simulink model "SOC_Estimation_EKF"  (R2025b)
settings: Solver=FixedStepDiscrete  StartTime=0.0  StopTime=10000  FixedStep=0.1  RelTol=1e-3
model workspace (MAT data in the model file):
  R = 20
  Rmn = 0.0008432
  Ts = 0.2
libraries: BatteryEstimators x1
settings Model: Creator=HP  LastModifiedBy=HP

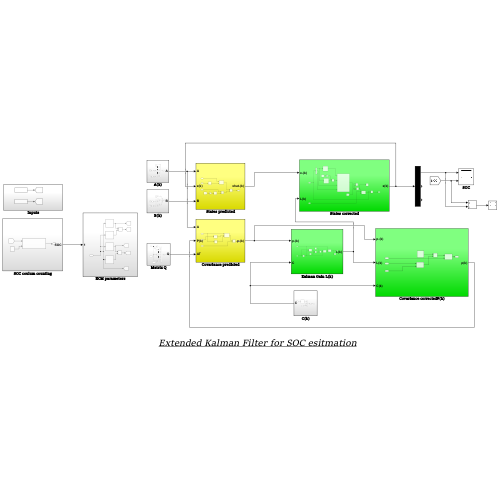
[thumbnail: Simulink's stored preview of the top-level diagram]
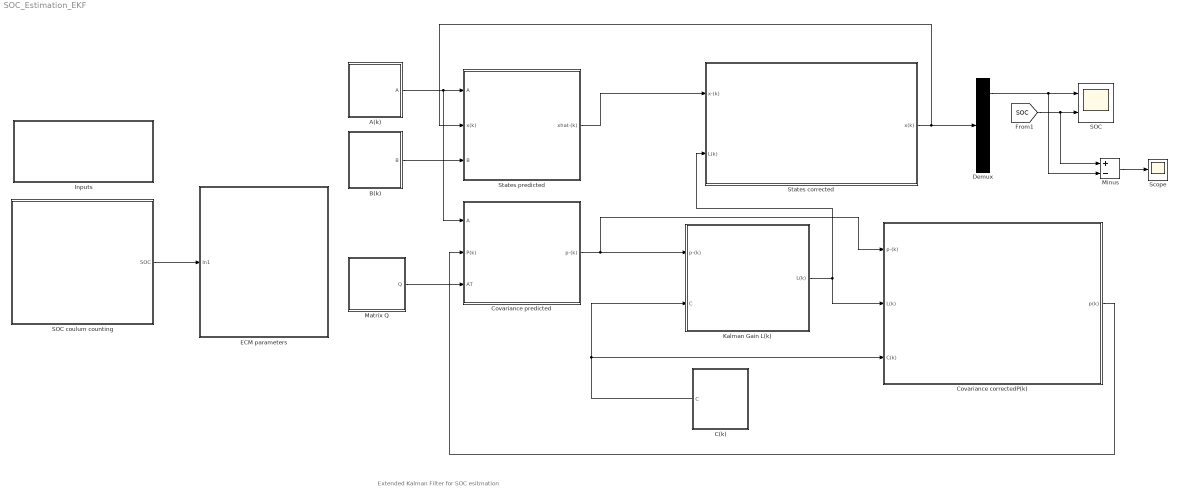
== system SOC_Estimation_EKF ==
  note: Extended Kalman Filter for SOC esitmation
  A(k) : Subsystem
  B(k) : Subsystem
  C(k) : Subsystem
  Covariance correctedP(k) : Subsystem
  Covariance predicted : Subsystem
  Demux : Demux  Outputs=3
  ECM parameters : Subsystem
  Inputs : Subsystem
  Kalman Gain L(k) : Subsystem
  Matrix Q : Subsystem
  Minus : Sum  Inputs=+-
  SOC : Scope  NumInputPorts=2
      settings: ActiveDisplayYMinimum=-0.11556307804743458  ActiveDisplayYMaximum=1.1239514531163817
  SOC coulum counting : Subsystem
  Scope : Scope
      settings: ActiveDisplayYMinimum=-0.040133146008147769  ActiveDisplayYMaximum=0.033848860038154627  DataLoggingVariableName=ScopeData4
  States corrected : Subsystem
  States predicted : Subsystem
  wires:
  A(k)/1(A) -> States predicted/1(A), Covariance predicted/1(A)
  B(k)/1(B) -> States predicted/3(B)
  Matrix Q/1(Q) -> Covariance predicted/3(AT)
  Covariance predicted/1(p-(k)) -> Kalman Gain L(k)/1(p-(k)), Covariance correctedP(k)/1(p-(k))
  C(k)/1(C) -> Kalman Gain L(k)/2(C), Covariance correctedP(k)/3(C(k))
  Kalman Gain L(k)/1(L(k)) -> States corrected/2(L(k)), Covariance correctedP(k)/2(L(k))
  Covariance correctedP(k)/1(p(k)) -> Covariance predicted/2(P(k))
  States predicted/1(xhat-(k)) -> States corrected/1(x-(k))
  States corrected/1(x(k)) -> States predicted/2(x(k)), Demux/1
  Demux/1 -> Minus/2, SOC/1
  [SOC] -> Minus/1, SOC/2
  SOC coulum counting/1(SOC) -> ECM parameters/1(In1)
  Minus/1 -> Scope/1

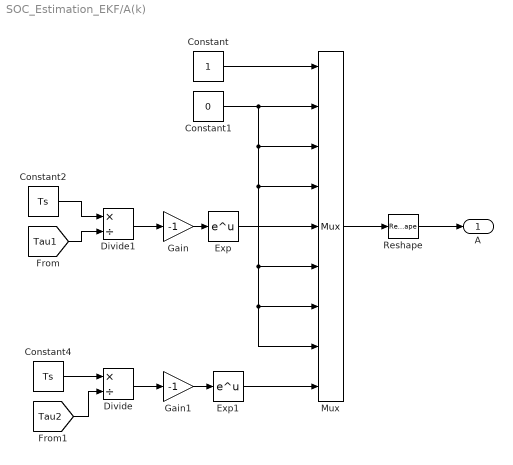
== system SOC_Estimation_EKF/A(k) ==
  Constant : Constant
  Constant1 : Constant  Value=0
  Constant2 : Constant  Value=Ts
  Constant4 : Constant  Value=Ts
  Divide : Product  Inputs=*/
  Divide1 : Product  Inputs=*/
  Exp : Math
  Exp1 : Math
  Gain : Gain  Gain=-1
  Gain1 : Gain  Gain=-1
  Mux : Mux  Inputs=9
  Reshape : Reshape  OutputDimensionality=Customize  OutputDimensions=[3,3]
  A : Outport
  wires:
  Constant1/1 -> Mux/6, Mux/7, Mux/8, Mux/4, Mux/3, Mux/2
  Constant4/1 -> Divide/1
  Constant/1 -> Mux/1
  [Tau2] -> Divide/2
  Divide1/1 -> Gain/1
  Gain1/1 -> Exp1/1
  Gain/1 -> Exp/1
  Divide/1 -> Gain1/1
  Constant2/1 -> Divide1/1
  [Tau1] -> Divide1/2
  Mux/1 -> Reshape/1
  Reshape/1 -> A/1
  Exp/1 -> Mux/5
  Exp1/1 -> Mux/9

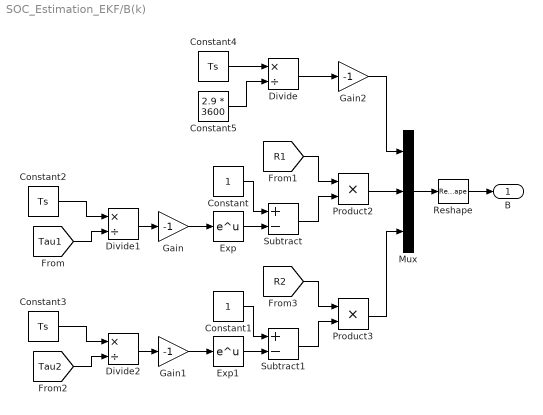
== system SOC_Estimation_EKF/B(k) ==
  Constant : Constant
  Constant1 : Constant
  Constant2 : Constant  Value=Ts
  Constant3 : Constant  Value=Ts
  Constant4 : Constant  Value=Ts
  Constant5 : Constant  Value=2.9 * 3600
  Divide : Product  Inputs=*/
  Divide1 : Product  Inputs=*/
  Divide2 : Product  Inputs=*/
  Exp : Math
  Exp1 : Math
  Gain : Gain  Gain=-1
  Gain1 : Gain  Gain=-1
  Gain2 : Gain  Gain=-1
  Mux : Mux  Inputs=3
  Product2 : Product
  Product3 : Product
  Reshape : Reshape  OutputDimensionality=Customize  OutputDimensions=[3,1]
  Subtract : Sum  Inputs=+-
  Subtract1 : Sum  Inputs=+-
  B : Outport
  wires:
  Product3/1 -> Mux/3
  Gain/1 -> Exp/1
  Constant3/1 -> Divide2/1
  [R2] -> Product3/1
  Constant/1 -> Subtract/1
  Divide/1 -> Gain2/1
  Gain2/1 -> Mux/1
  Subtract1/1 -> Product3/2
  Divide2/1 -> Gain1/1
  [Tau2] -> Divide2/2
  Gain1/1 -> Exp1/1
  Constant1/1 -> Subtract1/1
  Constant5/1 -> Divide/2
  Exp1/1 -> Subtract1/2
  Constant2/1 -> Divide1/1
  [Tau1] -> Divide1/2
  Divide1/1 -> Gain/1
  [R1] -> Product2/1
  Constant4/1 -> Divide/1
  Product2/1 -> Mux/2
  Subtract/1 -> Product2/2
  Mux/1 -> Reshape/1
  Exp/1 -> Subtract/2
  Reshape/1 -> B/1

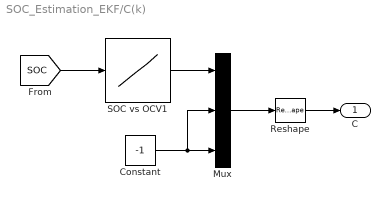
== system SOC_Estimation_EKF/C(k) ==
  Constant : Constant  Value=-1
  Mux : Mux  Inputs=3
  Reshape : Reshape  OutputDimensionality=Customize  OutputDimensions=[1,3]
  SOC vs OCV1 : Lookup_n-D  NumberOfTableDimensions=1  BreakpointsForDimension1=[0;0.017000000000000001;0.034000000000000002;0.050999999999999997;0.068000000000000005;0.085000000000000006;0.10199999999999999;0.11899999999999999;0.13600000000000001;0.152;0.16900000000000001;0.186;0.20300000000000001;0.22;0.23699999999999999;0.254;0.27100000000000002;0.28799999999999998;0.30499999999999999;0.32200000000000001;0.33900000000000002;0.35599999999999998;0.373;0.39000000000000001;0.40699999999999997;0.42399999999999999;0.441;0.45800000000000002;0.47499999999999998;0.49199999999999999;0.50800000000000001;0.52500000000000002;0.54200000000000004;0.55900000000000005;0.57599999999999996;0.59299999999999997;0.60999999999999999;0.627;0.64400000000000002;0.66100000000000003;0.67800000000000005;0.69499999999999995;0.71199999999999997;0.72899999999999998;0.746;0.76300000000000001;0.78000000000000003;0.79700000000000004;0.81399999999999995;0.82999999999999996;0.84699999999999998;0.86399999999999999;0.88100000000000001;0.89800000000000002;0.91500000000000004;0.93200000000000005;0.94899999999999995;0.96599999999999997;0.98299999999999998;1]  BreakpointsForDimension3=[5, 7]  Table=[32.28235294;20.56764706;6.15294118;2.68235294;1.62647059;1.24705882;1.28529412;1.43823529;1.42352941;1.32647059;1.17352941;1.05882353;1.05882353;1.00588235;0.89117647;0.79411765;0.71764706;0.66176471;0.60588235;0.56764706;0.56764706;0.56764706;0.5470588199999999;0.56764706;0.56764706;0.56764706;0.58823529;0.66176471;0.6882352900000001;0.67352941;0.7647058799999999;0.89117647;1.02352941;1.13823529;1.17352941;1.10882353;0.99117647;0.94705882;0.90882353;0.86470588;0.8441176500000001;0.83235294;0.81470588;0.79411765;0.79411765;0.82352941;0.90882353;0.97352941;1.00588235;1.02058824;1.11764706;1.22647059;1.10294118;0.97941176;0.87352941;0.79411765;0.79411765;1.00588235;1.30294118;1.4]  InternalRulePriority=Speed  RndMeth=Simplest
  C : Outport
  wires:
  SOC vs OCV1/1 -> Mux/1
  Constant/1 -> Mux/2, Mux/3
  [SOC] -> SOC vs OCV1/1
  Mux/1 -> Reshape/1
  Reshape/1 -> C/1

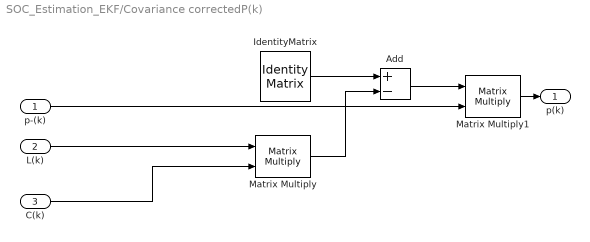
== system SOC_Estimation_EKF/Covariance correctedP(k) ==
  p-(k) : Inport
  L(k) : Inport  Port=2
  C(k) : Inport  Port=3
  Add : Sum  Inputs=+-
  IdentityMatrix : IdentityMatrix  OutputDimensions=3
  Matrix Multiply : Product  Multiplication=Matrix(*)
  Matrix Multiply1 : Product  Multiplication=Matrix(*)
  p(k) : Outport
  wires:
  Matrix Multiply/1 -> Add/2
  L(k)/1 -> Matrix Multiply/1
  p-(k)/1 -> Matrix Multiply1/2
  C(k)/1 -> Matrix Multiply/2
  IdentityMatrix/1 -> Add/1
  Add/1 -> Matrix Multiply1/1
  Matrix Multiply1/1 -> p(k)/1

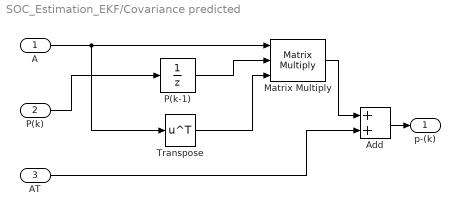
== system SOC_Estimation_EKF/Covariance predicted ==
  A : Inport
  P(k) : Inport  Port=2
  AT : Inport  Port=3
  Add : Sum
  Matrix Multiply : Product  Inputs=3  Multiplication=Matrix(*)
  P(k-1) : UnitDelay  SampleTime=-1  HasFrameUpgradeWarning=on
  Transpose : Math  Operator=transpose
  p-(k) : Outport
  wires:
  P(k)/1 -> P(k-1)/1
  A/1 -> Matrix Multiply/1, Transpose/1
  P(k-1)/1 -> Matrix Multiply/2
  AT/1 -> Add/2
  Transpose/1 -> Matrix Multiply/3
  Add/1 -> p-(k)/1
  Matrix Multiply/1 -> Add/1

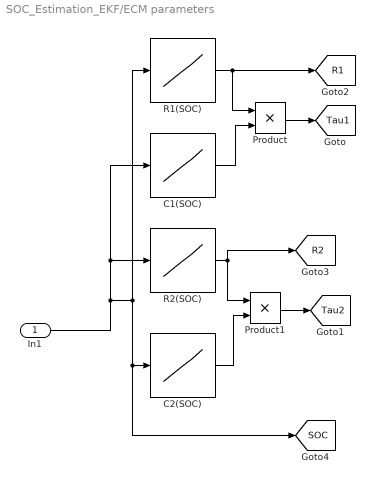
== system SOC_Estimation_EKF/ECM parameters ==
  In1 : Inport
  C1(SOC) : Lookup_n-D  NumberOfTableDimensions=1  BreakpointsForDimension1=[0.045807;0.04861;0.049997;0.09027200000000001;0.095828;0.098607;0.099993;0.14024;0.1458;0.14861;0.15;0.17914;0.19025;0.1958;0.19861;0.19999;0.22914;0.24025;0.24581;0.24861;0.25;0.27914;0.29025;0.29581;0.29861;0.3;0.37915;0.39027;0.39583;0.3986;0.39999;0.47914;0.49025;0.4958;0.49861;0.49999;0.57917;0.59027;0.59583;0.59861;0.67913;0.69025;0.69581;0.69861;0.7;0.7791400000000001;0.79025;0.79581;0.79861;0.8;0.87904;0.8902600000000001;0.8958199999999999;0.8986;0.9;0.92903;0.94025;0.94581;0.94861;0.95;0.97914;0.99026;0.99581;0.99861;1]  BreakpointsForDimension3=[5, 7]  Table=[9.757899999999999;10.71;19.27;9.6311;10.157;9.1839;7.5693;15.897;6.3554;7.6236;6.7393;7.7947;34.343;7.0897;6.9869;8.0646;10.291;128.49;9.2583;8.628;10.569;3.0789;34.161;8.1753;8.1843;13.019;10.1;46.123;9.795400000000001;11.091;15.634;8.213800000000001;31.921;9.789999999999999;10.357;12.364;15.812;507.21;15.291;17.025;4.9769;86.715;10.771;11.678;16.952;4.0064;71.312;13.377;14.851;17.855;16.185;258.83;9.310700000000001;12.325;12.739;12.404;193.01;11.32;10.578;11.323;10.955;21.418;8.9283;8.207800000000001;7.1378]  InternalRulePriority=Speed  RndMeth=Simplest
  C2(SOC) : Lookup_n-D  NumberOfTableDimensions=1  BreakpointsForDimension1=[0.045807;0.04861;0.049997;0.09027200000000001;0.095828;0.098607;0.099993;0.14024;0.1458;0.14861;0.15;0.17914;0.19025;0.1958;0.19861;0.19999;0.22914;0.24025;0.24581;0.24861;0.25;0.27914;0.29025;0.29581;0.29861;0.3;0.37915;0.39027;0.39583;0.3986;0.39999;0.47914;0.49025;0.4958;0.49861;0.49999;0.57917;0.59027;0.59583;0.59861;0.67913;0.69025;0.69581;0.69861;0.7;0.7791400000000001;0.79025;0.79581;0.79861;0.8;0.87904;0.8902600000000001;0.8958199999999999;0.8986;0.9;0.92903;0.94025;0.94581;0.94861;0.95;0.97914;0.99026;0.99581;0.99861;1]  BreakpointsForDimension3=[5, 7]  Table=[28.27;165.16;320.69;27.712;253.09;392.4;484.26;286.89;667.1;797.24;821.7;276.23;791.1799999999999;900.02;867.21;982.5599999999999;578.61;1042.4;1006.1;1040.2;960.4;789.21;1030.3;1069;1066.3;989.14;721.55;1138.1;1129.9;1119.4;1161;707.97;1170;1131;1148.4;1135.7;1346.9;2263.1;1223.3;986.53;635.45;1463;1017.1;802.7;751.76;689.47;1290.9;949.45;785.04;766.98;1784.1;1291.1;899.59;822.66;797.77;996.24;1271;972.37;906.33;953.26;1063;1097.7;990.14;909.11;837.3200000000001]  InternalRulePriority=Speed  RndMeth=Simplest
  Product : Product
  Product1 : Product
  R1(SOC) : Lookup_n-D  NumberOfTableDimensions=1  BreakpointsForDimension1=[0.045807;0.04861;0.049997;0.09027200000000001;0.095828;0.098607;0.099993;0.14024;0.1458;0.14861;0.15;0.17914;0.19025;0.1958;0.19861;0.19999;0.22914;0.24025;0.24581;0.24861;0.25;0.27914;0.29025;0.29581;0.29861;0.3;0.37915;0.39027;0.39583;0.3986;0.39999;0.47914;0.49025;0.4958;0.49861;0.49999;0.57917;0.59027;0.59583;0.59861;0.67913;0.69025;0.69581;0.69861;0.7;0.7791400000000001;0.79025;0.79581;0.79861;0.8;0.87904;0.8902600000000001;0.8958199999999999;0.8986;0.9;0.92903;0.94025;0.94581;0.94861;0.95;0.97914;0.99026;0.99581;0.99861;1]  BreakpointsForDimension3=[5, 7]  Table=[0.037938;0.076447;0.11612;0.037632;0.056353;0.048597;0.045211;0.02245;0.026899;0.021454;0.021757;0.026914;0.0077714;0.016485;0.015735;0.014616;0.021046;0.004533;0.012247;0.01283;0.012104;0.019173;0.0058875;0.012706;0.013166;0.011323;0.017322;0.0052329;0.011749;0.010926;0.009813000000000001;0.016731;0.0060175;0.011748;0.011411;0.010247;0.018135;0.0042689;0.010879;0.011984;0.016336;0.0056556;0.012305;0.013495;0.012597;0.016561;0.0055684;0.010945;0.012297;0.012084;0.019124;0.0042543;0.013181;0.012843;0.012765;0.018586;0.0045275;0.011688;0.013391;0.013777;0.01955;0.007903200000000001;0.014133;0.015549;0.015915]  InternalRulePriority=Speed  RndMeth=Simplest
  R2(SOC) : Lookup_n-D  NumberOfTableDimensions=1  BreakpointsForDimension1=[0.045807;0.04861;0.049997;0.09027200000000001;0.095828;0.098607;0.099993;0.14024;0.1458;0.14861;0.15;0.17914;0.19025;0.1958;0.19861;0.19999;0.22914;0.24025;0.24581;0.24861;0.25;0.27914;0.29025;0.29581;0.29861;0.3;0.37915;0.39027;0.39583;0.3986;0.39999;0.47914;0.49025;0.4958;0.49861;0.49999;0.57917;0.59027;0.59583;0.59861;0.67913;0.69025;0.69581;0.69861;0.7;0.7791400000000001;0.79025;0.79581;0.79861;0.8;0.87904;0.8902600000000001;0.8958199999999999;0.8986;0.9;0.92903;0.94025;0.94581;0.94861;0.95;0.97914;0.99026;0.99581;0.99861;1]  BreakpointsForDimension3=[5, 7]  Table=[0.071321;0.089744;0.047068;0.028716;0.081313;0.051312;0.044524;0.071516;0.025727;0.025386;0.02597;0.067118;0.029108;0.024102;0.026335;0.025064;0.035581;0.02348;0.021914;0.022956;0.028735;0.027004;0.022795;0.022925;0.023911;0.034644;0.014599;0.019644;0.019234;0.021182;0.021771;0.011275;0.015597;0.016874;0.018573;0.019889;0.01001;0.020546;0.024649;0.033802;0.012282;0.027028;0.026501;0.028818;0.032779;0.012322;0.022938;0.022283;0.024856;0.026474;0.0099907;0.020073;0.018904;0.02035;0.022573;0.015395;0.017126;0.016158;0.017248;0.019725;0.011255;0.014583;0.017596;0.020712;0.02094]  InternalRulePriority=Speed  RndMeth=Simplest
  tag scope: R1=global, R2=global, SOC=global, Tau1=global, Tau2=global
  wires:
  C2(SOC)/1 -> Product1/2
  Product/1 -> [Tau1]
  R1(SOC)/1 -> Product/1, [R1]
  In1/1 -> [SOC], C2(SOC)/1, R1(SOC)/1, C1(SOC)/1, R2(SOC)/1
  Product1/1 -> [Tau2]
  C1(SOC)/1 -> Product/2
  R2(SOC)/1 -> Product1/1, [R2]

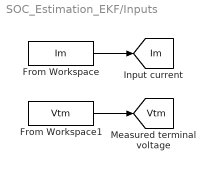
== system SOC_Estimation_EKF/Inputs ==
  From Workspace : FromWorkspace  VariableName=Im  SampleTime=-1
  From Workspace1 : FromWorkspace  VariableName=Vtm  SampleTime=-1
  tag scope: Im=global, Vtm=global
  wires:
  From Workspace/1 -> [Im]
  From Workspace1/1 -> [Vtm]

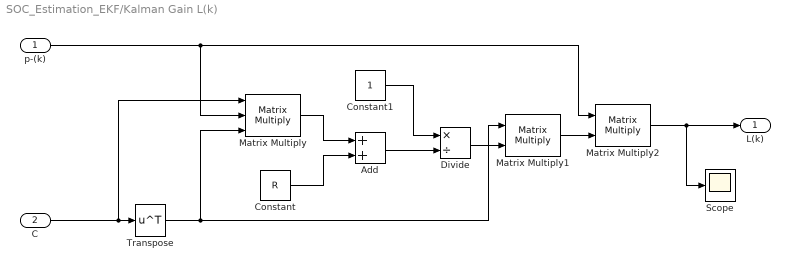
== system SOC_Estimation_EKF/Kalman Gain L(k) ==
  p-(k) : Inport
  C : Inport  Port=2
  Add : Sum
  Constant : Constant  Value=R
  Constant1 : Constant
  Divide : Product  Inputs=*/
  Matrix Multiply : Product  Inputs=3  Multiplication=Matrix(*)
  Matrix Multiply1 : Product  Multiplication=Matrix(*)
  Matrix Multiply2 : Product  Multiplication=Matrix(*)
  Scope : Scope
      settings: ActiveDisplayYMinimum=-0.015675362785877577  ActiveDisplayYMaximum=0.11185033850037487  DataLoggingVariableName=ScopeData3
  Transpose : Math  Operator=transpose
  L(k) : Outport
  wires:
  Matrix Multiply1/1 -> Matrix Multiply2/2
  Transpose/1 -> Matrix Multiply1/1, Matrix Multiply/3
  Divide/1 -> Matrix Multiply1/2
  C/1 -> Matrix Multiply/1, Transpose/1
  Matrix Multiply/1 -> Add/1
  Constant/1 -> Add/2
  p-(k)/1 -> Matrix Multiply2/1, Matrix Multiply/2
  Add/1 -> Divide/2
  Constant1/1 -> Divide/1
  Matrix Multiply2/1 -> Scope/1, L(k)/1

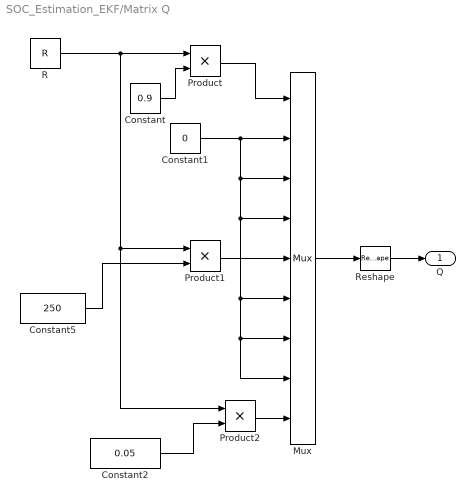
== system SOC_Estimation_EKF/Matrix Q ==
  Constant : Constant  Value=0.9
  Constant1 : Constant  Value=0
  Constant2 : Constant  Value=0.05
  Constant5 : Constant  Value=250
  Mux : Mux  Inputs=9
  Product : Product
  Product1 : Product
  Product2 : Product
  R : Constant  Value=R
  Reshape : Reshape  OutputDimensionality=Customize  OutputDimensions=[3,3]
  Q : Outport
  wires:
  Constant1/1 -> Mux/2, Mux/3, Mux/4, Mux/8, Mux/7, Mux/6
  Product1/1 -> Mux/5
  Product2/1 -> Mux/9
  Mux/1 -> Reshape/1
  Reshape/1 -> Q/1
  Constant/1 -> Product/2
  Product/1 -> Mux/1
  Constant5/1 -> Product1/2
  Constant2/1 -> Product2/2
  R/1 -> Product1/1, Product2/1, Product/1

== system SOC_Estimation_EKF/SOC coulum counting ==
  Constant : Constant
  SOC Estimator (Coulomb Counting) : BatteryEstimators/SOC Estimator (Coulomb Counting)  CurrentInputPartition=on  AH=2.9  Ts=-1  DataType=Inherit: auto
      settings: LibrarySourceBlock=|
      | batt_sl_lib/Estimators/SOC Estimator
      | (Coulomb Counting)
  SOC : Outport
  wires:
  SOC Estimator (Coulomb Counting)/1 -> SOC/1
  Constant/1 -> SOC Estimator (Coulomb Counting)/2
  [Im] -> SOC Estimator (Coulomb Counting)/1

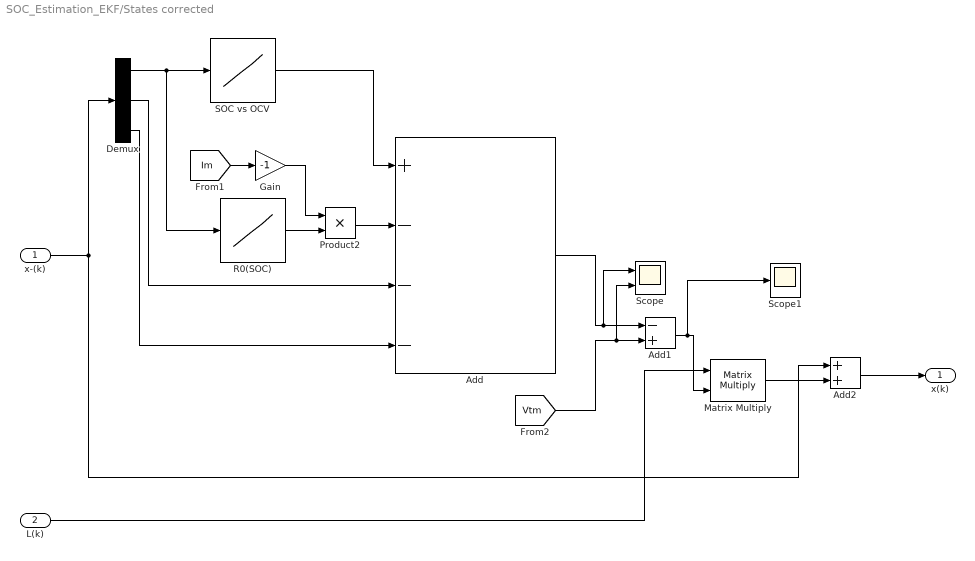
== system SOC_Estimation_EKF/States corrected ==
  x-(k) : Inport
  L(k) : Inport  Port=2
  Add : Sum  Inputs=+---
  Add1 : Sum  Inputs=-+
  Add2 : Sum
  Demux : Demux  Outputs=3
  Gain : Gain  Gain=-1
  Matrix Multiply : Product  Multiplication=Matrix(*)
  Product2 : Product
  R0(SOC) : Lookup_n-D  NumberOfTableDimensions=1  BreakpointsForDimension1=[0.045807;0.04861;0.049997;0.09027200000000001;0.095828;0.098607;0.099993;0.14024;0.1458;0.14861;0.15;0.17914;0.19025;0.1958;0.19861;0.19999;0.22914;0.24025;0.24581;0.24861;0.25;0.27914;0.29025;0.29581;0.29861;0.3;0.37915;0.39027;0.39583;0.3986;0.39999;0.47914;0.49025;0.4958;0.49861;0.49999;0.57917;0.59027;0.59583;0.59861;0.67913;0.69025;0.69581;0.69861;0.7;0.7791400000000001;0.79025;0.79581;0.79861;0.8;0.87904;0.8902600000000001;0.8958199999999999;0.8986;0.9;0.92903;0.94025;0.94581;0.94861;0.95;0.97914;0.99026;0.99581;0.99861;1]  BreakpointsForDimension3=[5, 7]  Table=[0.049075;0.025722;0.026458;0.046408;0.0249;0.027929;0.025798;0.032516;0.023069;0.025835;0.023545;0.037074;0.031878;0.021418;0.021384;0.022184;0.03225;0.030131;0.021533;0.020726;0.021473;0.029993;0.026582;0.019435;0.018941;0.02098;0.028423;0.025805;0.018933;0.019833;0.021195;0.027588;0.024253;0.018327;0.018935;0.019882;0.027443;0.027386;0.019996;0.019732;0.027407;0.025473;0.018656;0.018395;0.019906;0.027518;0.025612;0.02027;0.019947;0.020796;0.028239;0.028302;0.01933;0.020731;0.021222;0.02905;0.029273;0.022486;0.021851;0.021942;0.030344;0.02786;0.023522;0.02362;0.024004]  InternalRulePriority=Speed  RndMeth=Simplest
  SOC vs OCV : Lookup_n-D  NumberOfTableDimensions=1  BreakpointsForDimension1=[0;0.017000000000000001;0.034000000000000002;0.050999999999999997;0.068000000000000005;0.085000000000000006;0.10199999999999999;0.11899999999999999;0.13600000000000001;0.152;0.16900000000000001;0.186;0.20300000000000001;0.22;0.23699999999999999;0.254;0.27100000000000002;0.28799999999999998;0.30499999999999999;0.32200000000000001;0.33900000000000002;0.35599999999999998;0.373;0.39000000000000001;0.40699999999999997;0.42399999999999999;0.441;0.45800000000000002;0.47499999999999998;0.49199999999999999;0.50800000000000001;0.52500000000000002;0.54200000000000004;0.55900000000000005;0.57599999999999996;0.59299999999999997;0.60999999999999999;0.627;0.64400000000000002;0.66100000000000003;0.67800000000000005;0.69499999999999995;0.71199999999999997;0.72899999999999998;0.746;0.76300000000000001;0.78000000000000003;0.79700000000000004;0.81399999999999995;0.82999999999999996;0.84699999999999998;0.86399999999999999;0.88100000000000001;0.89800000000000002;0.91500000000000004;0.93200000000000005;0.94899999999999995;0.96599999999999997;0.98299999999999998;1]  BreakpointsForDimension3=[5, 7]  Table=[2.4995;3.0483;3.1988;3.2574;3.2902;3.3127;3.3326;3.3564;3.3815;3.4047;3.4266;3.4446;3.4626;3.4806;3.4967;3.5109;3.5237;3.5353;3.5462;3.5559;3.5655;3.5752;3.5848;3.5938;3.6035;3.6131;3.6228;3.6331;3.6453;3.6562;3.6685;3.6826;3.6987;3.7174;3.7373;3.7573;3.7746;3.7907;3.8068;3.8216;3.8364;3.8505;3.8647;3.8782;3.8917;3.9052;3.9207;3.9361;3.9528;3.9696;3.9876;4.0069;4.0262;4.0442;4.0596;4.0738;4.0867;4.1008;4.1201;4.1439]  InternalRulePriority=Speed  RndMeth=Simplest
  Scope : Scope  NumInputPorts=2
      settings: ActiveDisplayYMinimum=1.40156552815179  ActiveDisplayYMaximum=4.57251713483082
  Scope1 : Scope
      settings: ActiveDisplayYMinimum=-0.13988247870906267  ActiveDisplayYMaximum=0.14925645013148925  DataLoggingVariableName=ScopeData2
  x(k) : Outport
  wires:
  Demux/2 -> Add/3
  R0(SOC)/1 -> Product2/2
  x-(k)/1 -> Add2/1, Demux/1
  Product2/1 -> Add/2
  [Vtm] -> Scope/2, Add1/2
  Gain/1 -> Product2/1
  Demux/1 -> R0(SOC)/1, SOC vs OCV/1
  [Im] -> Gain/1
  SOC vs OCV/1 -> Add/1
  Add/1 -> Scope/1, Add1/1
  Demux/3 -> Add/4
  Matrix Multiply/1 -> Add2/2
  Add2/1 -> x(k)/1
  Add1/1 -> Scope1/1, Matrix Multiply/2
  L(k)/1 -> Matrix Multiply/1

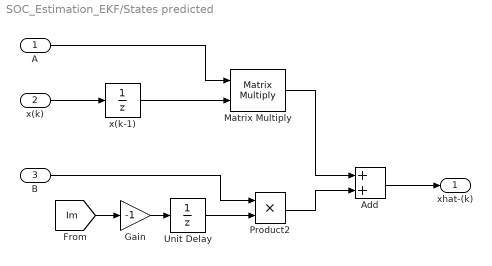
== system SOC_Estimation_EKF/States predicted ==
  A : Inport
  x(k) : Inport  Port=2
  B : Inport  Port=3
  Add : Sum
  Gain : Gain  Gain=-1
  Matrix Multiply : Product  Multiplication=Matrix(*)
  Product2 : Product
  Unit Delay : UnitDelay  SampleTime=-1  HasFrameUpgradeWarning=on
  x(k-1) : UnitDelay  SampleTime=-1  HasFrameUpgradeWarning=on
  xhat-(k) : Outport
  wires:
  A/1 -> Matrix Multiply/1
  x(k-1)/1 -> Matrix Multiply/2
  Add/1 -> xhat-(k)/1
  Unit Delay/1 -> Product2/2
  [Im] -> Gain/1
  Product2/1 -> Add/2
  B/1 -> Product2/1
  Matrix Multiply/1 -> Add/1
  x(k)/1 -> x(k-1)/1
  Gain/1 -> Unit Delay/1
